simulink model "dqc_debugging"  (Simulink 7.9)
settings: Solver=ode45  StartTime=0.0  StopTime=inf  RelTol=1e-3
libraries: utility x1
settings Model: Creator=jorhabib  LastModifiedBy=jorhabib

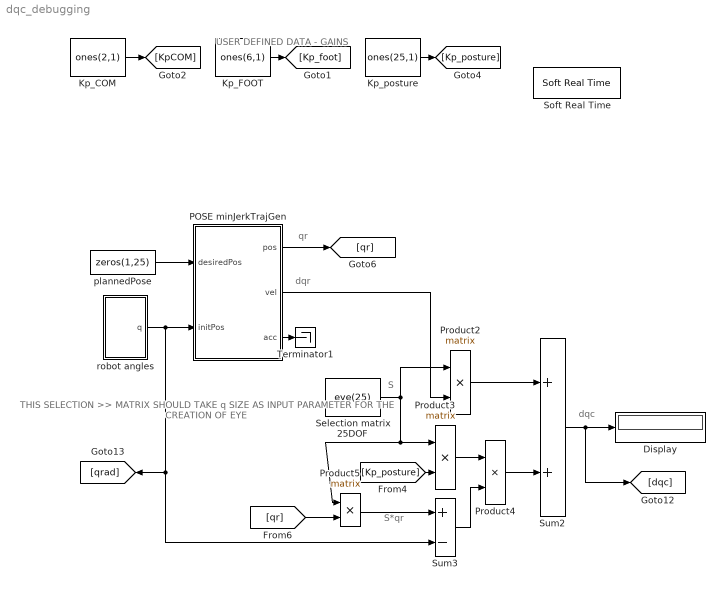
== system dqc_debugging ==
  note: qr
  note: dqr
  note: S
  note: dqc
  note: S*qr
  note: THIS SELECTION    >>
      | MATRIX SHOULD
      | TAKE q SIZE AS
      | INPUT PARAMETER
      | FOR THE CREATION
      | OF EYE
  note: USER DEFINED DATA - GAINS
  Display : Display
  Kp_COM : Constant  Value=ones(2,1)
  Kp_FOOT : Constant  Value=ones(6,1)
  Kp_posture : Constant  Value=ones(25,1)
  POSE minJerkTrajGen : Subsystem
  Product2 : Product  Multiplication=Matrix(*)  RndMeth=Zero
  Product3 : Product  Multiplication=Matrix(*)  RndMeth=Zero
  Product4 : Product  RndMeth=Zero
  Product5 : Product  Multiplication=Matrix(*)  RndMeth=Zero
  Selection matrix 25DOF : Constant  Value=eye(25)
  Soft Real Time : utility/Soft Real Time  x=0.1
  Sum2 : Sum
  Sum3 : Sum  Inputs=+-
  Terminator1 : Terminator
  plannedPose : Constant  Value=zeros(1,25)
  robot angles : Subsystem
  wires:
  robot angles/1(q) -> [qrad], Sum3/2, POSE minJerkTrajGen/2(initPos)
  plannedPose/1 -> POSE minJerkTrajGen/1(desiredPos)
  Selection matrix 25DOF/1 -> Product2/1, Product5/1, Product3/1
  Product2/1 -> Sum2/1
  [Kp_posture] -> Product3/2
  Product3/1 -> Product4/1
  Sum3/1 -> Product4/2
  Product4/1 -> Sum2/2
  Sum2/1 -> [dqc], Display/1
  Product5/1 -> Sum3/1
  POSE minJerkTrajGen/3(acc) -> Terminator1/1
  POSE minJerkTrajGen/1(pos) -> [qr]
  [qr] -> Product5/2
  POSE minJerkTrajGen/2(vel) -> Product2/2
  Kp_COM/1 -> [KpCOM]
  Kp_FOOT/1 -> [Kp_foot]
  Kp_posture/1 -> [Kp_posture]

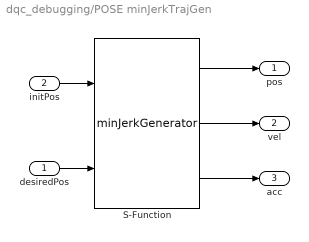
== system dqc_debugging/POSE minJerkTrajGen ==
  desiredPos : Inport
  initPos : Inport  Port=2
  S-Function : S-Function  FunctionName=minJerkGenerator  Parameters=dim, rate, tt  EnableBusSupport=off  mask{dim=25, rate=10, tt=4}
      mask prompts: dim "Trajectory dimension (int)"; rate "Simulation rate (int) [ms]"; tt "Trajectory time [s]"
  pos : Outport
  vel : Outport  Port=2
  acc : Outport  Port=3
  wires:
  desiredPos/1 -> S-Function/2
  initPos/1 -> S-Function/1
  S-Function/3 -> acc/1
  S-Function/1 -> pos/1
  S-Function/2 -> vel/1

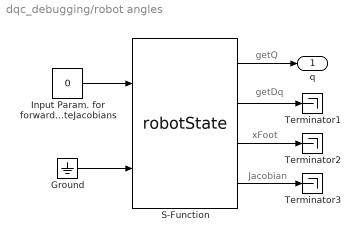
== system dqc_debugging/robot angles ==
  note: getDq
  note: xFoot
  note: getQ
  note: Jacobian
  Ground : Ground
  "Input Param. for forwardKinematics and  computeJacobians " : Constant  Value=0  OutDataTypeStr=int8
  S-Function : S-Function  FunctionName=robotState  Parameters=val,robotname,localname  EnableBusSupport=off  mask{val=0, robotname='icubSim', localname='robotState'}
      mask prompts: val "Value"; robotname "Robot Name (icub - icubSim)"; localname "Module Name"
  Terminator1 : Terminator
  Terminator2 : Terminator
  Terminator3 : Terminator
  q : Outport
  wires:
  Ground/1 -> S-Function/2
  S-Function/2 -> Terminator1/1
  S-Function/1 -> q/1
  S-Function/3 -> Terminator2/1
  "Input Param. for forwardKinematics and  computeJacobians "/1 -> S-Function/1
  S-Function/4 -> Terminator3/1
